simulink model "Unicorn_Demo1"  (R2015a)
settings: Solver=FixedStepDiscrete  StartTime=0.0  StopTime=10  RelTol=1e-3
undefined symbols (not defined in the file): UN
libraries: UnicornLib x1
settings Model: Creator=reitner  LastModifiedBy=walchshofer
settings DebuggingCC: FrameProcessingCompatibilityMsg=none

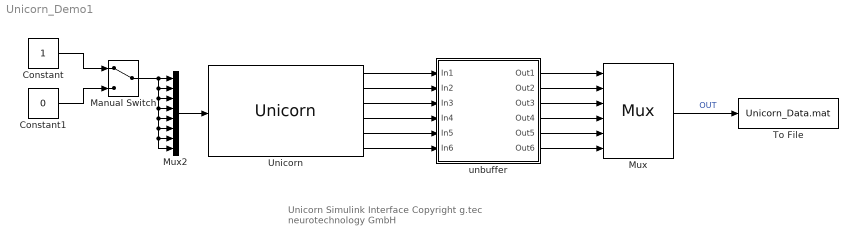
== system Unicorn_Demo1 ==
  note: Unicorn Simulink Interface
      | Copyright g.tec neurotechnology GmbH
  Constant : Constant  OutDataTypeStr=boolean
  Constant1 : Constant  Value=0  OutDataTypeStr=boolean
  Manual Switch : ManualSwitch
  Mux : Mux  Inputs=6
      settings: AttributesFormatString=multiplex
      mask Display:
      | port_label('input',1,'EEG')
      | port_label('input',2,'ACC')
      | port_label('input',3,'GYRO')
      | port_label('input',4,'VALID')
      | port_label('input',5,'BAT')
      | port_label('input',6,'CNT')
  Mux2 : Mux  Inputs=8
  To File : ToFile  Filename=Unicorn_Data.mat  MatrixName=y
  Unicorn : UnicornLib/Unicorn  serial=UN-2018.11.94  old_serial=UN-2018.11.94  frame_length=1  input_source=Electrode
  "unbuffer " : Subsystem
      mask Display:
      | port_label('input',1,'EEG')
      | port_label('input',2,'ACC')
      | port_label('input',3,'GYRO')
      | port_label('input',4,'VALID')
      | port_label('input',5,'BAT')
      | port_label('input',6,'CNT')
      | port_label('output',1,'EEG')
      | port_label('output',2,'ACC')
      | port_label('output',3,'GYRO')
      | port_label('output',4,'VALID')
      | port_label('output',5,'BAT')
      | port_label('output',6,'CNT')
  wires:
  Constant/1 -> Manual Switch/1
  Constant1/1 -> Manual Switch/2
  Unicorn/1 -> "unbuffer "/1(In1)
  Unicorn/2 -> "unbuffer "/2(In2)
  Unicorn/3 -> "unbuffer "/3(In3)
  Unicorn/4 -> "unbuffer "/4(In4)
  Unicorn/5 -> "unbuffer "/5(In5)
  Unicorn/6 -> "unbuffer "/6(In6)
  "unbuffer "/1(Out1) -> Mux/1
  "unbuffer "/2(Out2) -> Mux/2
  "unbuffer "/3(Out3) -> Mux/3
  "unbuffer "/4(Out4) -> Mux/4
  "unbuffer "/5(Out5) -> Mux/5
  "unbuffer "/6(Out6) -> Mux/6
  Mux/1 -> To File/1  "OUT"
  Mux2/1 -> Unicorn/1
  Manual Switch/1 -> Mux2/8, Mux2/7, Mux2/6, Mux2/5, Mux2/4, Mux2/3, Mux2/2, Mux2/1

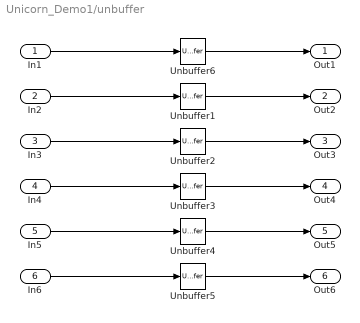
== system Unicorn_Demo1/unbuffer  ==
  In1 : Inport
  In2 : Inport  Port=2
  In3 : Inport  Port=3
  In4 : Inport  Port=4
  In5 : Inport  Port=5
  In6 : Inport  Port=6
  Unbuffer{1..6} (6 alike) : Unbuffer
  Out1 : Outport
  Out2 : Outport  Port=2
  Out3 : Outport  Port=3
  Out4 : Outport  Port=4
  Out5 : Outport  Port=5
  Out6 : Outport  Port=6
  wires:
  In1/1 -> Unbuffer6/1
  In6/1 -> Unbuffer5/1
  In2/1 -> Unbuffer1/1
  In3/1 -> Unbuffer2/1
  In4/1 -> Unbuffer3/1
  In5/1 -> Unbuffer4/1
  Unbuffer4/1 -> Out5/1
  Unbuffer5/1 -> Out6/1
  Unbuffer3/1 -> Out4/1
  Unbuffer2/1 -> Out3/1
  Unbuffer1/1 -> Out2/1
  Unbuffer6/1 -> Out1/1
